simulink model "kalman_model"  (R2018a)
settings: Solver=VariableStepAuto  StartTime=0.0  StopTime=ramp_new(end,1)  RelTol=1e-3
settings Model: Creator=adiravishankara  LastModifiedBy=adiravishankara

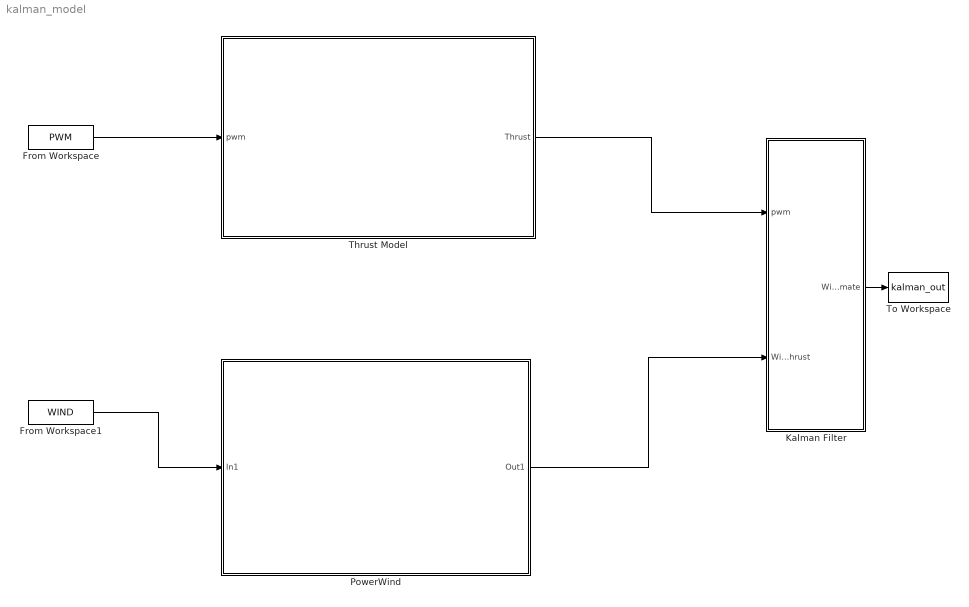
== system kalman_model ==
  From Workspace : FromWorkspace  VariableName=PWM  SampleTime=.01
  From Workspace1 : FromWorkspace  VariableName=WIND  SampleTime=.01
  Kalman Filter : Subsystem
  PowerWind : Subsystem
  Thrust Model : Subsystem
  To Workspace : ToWorkspace  VariableName=kalman_out  SampleTime=-1
  wires:
  From Workspace/1 -> Thrust Model/1(pwm)
  PowerWind/1(Out1) -> Kalman Filter/2(Wind_thrust)
  From Workspace1/1 -> PowerWind/1(In1)
  Thrust Model/1(Thrust) -> Kalman Filter/1(pwm)
  Kalman Filter/1(Wind estimate) -> To Workspace/1

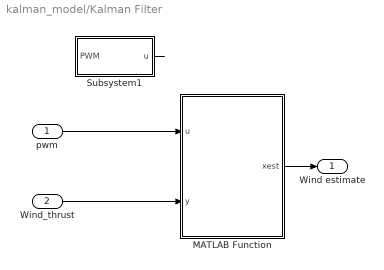
== system kalman_model/Kalman Filter ==
  pwm : Inport
  Wind_thrust : Inport  Port=2
  MATLAB Function : MATLAB Function  TreatAsAtomicUnit=on
  Subsystem1 : Subsystem
  Wind estimate : Outport
  wires:
  Subsystem1/1(u) -> ?
  Wind_thrust/1 -> MATLAB Function/2(y)
  pwm/1 -> MATLAB Function/1(u)
  MATLAB Function/1(xest) -> Wind estimate/1

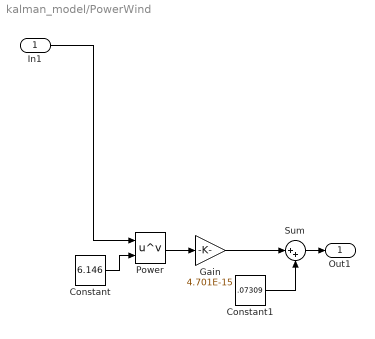
== system kalman_model/PowerWind ==
  In1 : Inport
  Constant : Constant  Value=6.146
  Constant1 : Constant  Value=.07309
  Gain : Gain  Gain=4.701E-15
  Power : Math  Operator=pow  SaturateOnIntegerOverflow=on
  Sum : Sum  Inputs=|++
  Out1 : Outport
  wires:
  Constant/1 -> Power/2
  Gain/1 -> Sum/1
  Sum/1 -> Out1/1
  In1/1 -> Power/1
  Power/1 -> Gain/1
  Constant1/1 -> Sum/2

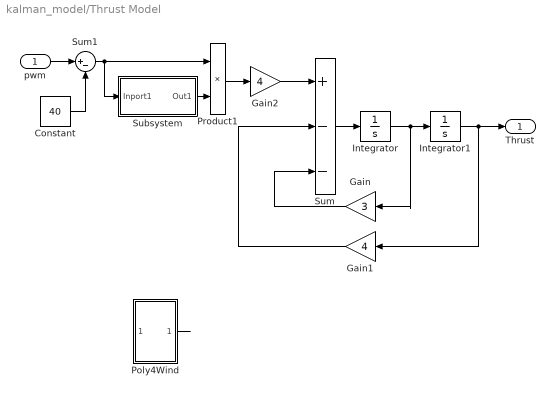
== system kalman_model/Thrust Model ==
  pwm : Inport
  Constant : Constant  Value=40
  Gain : Gain  Gain=3
  Gain1 : Gain  Gain=4
  Gain2 : Gain  Gain=4
  Integrator : Integrator
  Integrator1 : Integrator
  "Poly4Wind " : Subsystem
  Product1 : Product
  Subsystem : Subsystem
  Sum : Sum  Inputs=+--
  Sum1 : Sum  Inputs=|+-
  Thrust : Outport
  wires:
  Product1/1 -> Gain2/1
  Integrator/1 -> Gain/1, Integrator1/1
  Sum/1 -> Integrator/1
  Integrator1/1 -> Gain1/1, Thrust/1
  Gain/1 -> Sum/3
  Gain1/1 -> Sum/2
  Gain2/1 -> Sum/1
  "Poly4Wind "/1(Out1) -> ?
  pwm/1 -> Sum1/1
  Constant/1 -> Sum1/2
  Sum1/1 -> Subsystem/1(Inport1), Product1/1
  Subsystem/1(Out1) -> Product1/2

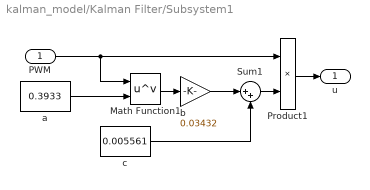
== system kalman_model/Kalman Filter/Subsystem1 ==
  PWM : Inport
  Math Function1 : Math  Operator=pow  SaturateOnIntegerOverflow=on
  Product1 : Product
  Sum1 : Sum  Inputs=|++
  a : Constant  Value=0.3933
  b : Gain  Gain=0.03432
  c : Constant  Value=0.005561
  u : Outport
  wires:
  Sum1/1 -> Product1/2
  Product1/1 -> u/1
  a/1 -> Math Function1/2
  b/1 -> Sum1/1
  PWM/1 -> Math Function1/1, Product1/1
  Math Function1/1 -> b/1
  c/1 -> Sum1/2

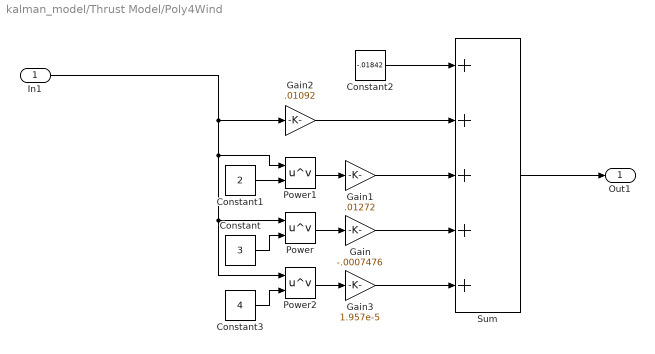
== system kalman_model/Thrust Model/Poly4Wind  ==
  In1 : Inport
  Constant : Constant  Value=3
  Constant1 : Constant  Value=2
  Constant2 : Constant  Value=-.01842
  Constant3 : Constant  Value=4
  Gain : Gain  Gain=-.0007476
  Gain1 : Gain  Gain=.01272
  Gain2 : Gain  Gain=.01092
  Gain3 : Gain  Gain=1.957e-5
  Power : Math  Operator=pow  SaturateOnIntegerOverflow=on
  Power1 : Math  Operator=pow  SaturateOnIntegerOverflow=on
  Power2 : Math  Operator=pow  SaturateOnIntegerOverflow=on
  Sum : Sum  Inputs=+++++
  Out1 : Outport
  wires:
  Gain/1 -> Sum/4
  Power/1 -> Gain/1
  Power1/1 -> Gain1/1
  In1/1 -> Power2/1, Power/1, Power1/1, Gain2/1
  Gain1/1 -> Sum/3
  Constant/1 -> Power/2
  Sum/1 -> Out1/1
  Gain2/1 -> Sum/2
  Constant1/1 -> Power1/2
  Constant2/1 -> Sum/1
  Constant3/1 -> Power2/2
  Power2/1 -> Gain3/1
  Gain3/1 -> Sum/5

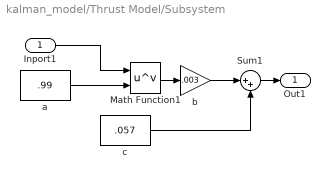
== system kalman_model/Thrust Model/Subsystem ==
  Inport1 : Inport
  Math Function1 : Math  Operator=pow  SaturateOnIntegerOverflow=on
  Sum1 : Sum  Inputs=|++
  a : Constant  Value=.99
  b : Gain  Gain=.003
  c : Constant  Value=.057
  Out1 : Outport
  wires:
  a/1 -> Math Function1/2
  b/1 -> Sum1/1
  Inport1/1 -> Math Function1/1
  Math Function1/1 -> b/1
  Sum1/1 -> Out1/1
  c/1 -> Sum1/2

== matlab function kalman_model/Kalman Filter/MATLAB Function ==
  settings: updateMethod=DISCRETE
  data: u input; xest output; y input
function xest  = fcn(u, y)
persistent P xh
if isempty(P)
    P = eye(2);
    xh = zeros(2,1);
end
% A = [0 1; -4 -3];
% B = [0; 4];
% C = [1 0];

Ad = [0.9998  0.009851; -0.0394    0.9702];
Bd = [0.000198; 0.0394];
Cd = [1 0];

Q = 1;
R = diag([5,5]);


% Model information
xh_bar = Ad * xh + Bd * u;
P_bar = Ad * P * Ad' + R;

% Measurement update
K = P_bar * Cd' * (Cd * P_bar * Cd' + Q)^-1;
xh = xh_bar + K * (y - Cd * xh_bar);
P = (1 - K * Cd) * P_bar;

xest = xh;
